simulink model "model_2_testform1"  (R2018a)
settings: Solver=VariableStepAuto  StartTime=0.0  StopTime=10.0  RelTol=1e-3
values from neighbouring files (symbols this model uses):
  Ad = [ 1   0     Tc        0 ... (first row only)    [vehicle_2DOF_model.m]    (also in vehicle_2DOF_model_2.m)
  Bd = [  0     0 ... (first row only)    [vehicle_2DOF_model.m]    (also in vehicle_2DOF_model_2.m)
  Fa = dlqr(Aa,Ba,Q,R)    [vehicle_2DOF_model.m]    (also in vehicle_2DOF_model_2.m = compute_Rstab_gain(ss(Aaug,Baug,Caug,zeros(2,2)), 2, pi/6, 5)
  Tc = 0.1    [vehicle_2DOF_model.m]    (also in vehicle_2DOF_model_2.m)
undefined symbols (not defined in the file or in its folder): DiscIntNeverNeededParam
settings Model: Creator=marwa  LastModifiedBy=marwa

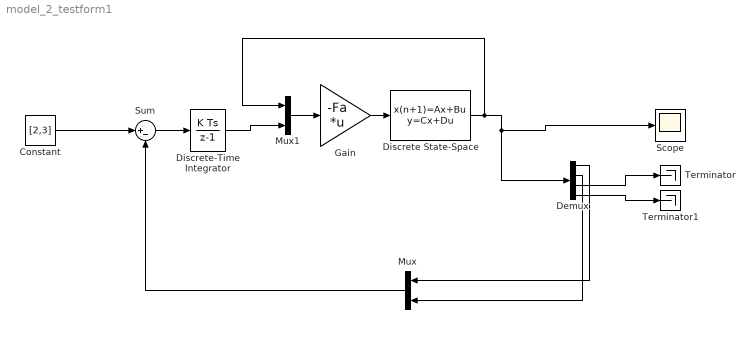
== system model_2_testform1 ==
  Constant : Constant  Value=[2,3]
  Demux : Demux
  Discrete State-Space : DiscreteStateSpace  A=Ad  B=Bd  C=eye(4)  D=zeros(4,2)  SampleTime=Tc
  Discrete-Time Integrator : DiscreteIntegrator  SampleTime=Tc  ICPrevOutput=DiscIntNeverNeededParam  ICPrevScaledInput=DiscIntNeverNeededParam
  Gain : Gain  Gain=-Fa  Multiplication=Matrix(K*u) (u vector)
  Mux : Mux  Inputs=2
  Mux1 : Mux  Inputs=2
  Scope : Scope
  Sum : Sum  Inputs=|+-
  Terminator : Terminator
  Terminator1 : Terminator
  wires:
  Constant/1 -> Sum/1
  Discrete State-Space/1 -> Mux1/1, Demux/1, Scope/1
  Sum/1 -> Discrete-Time Integrator/1
  Discrete-Time Integrator/1 -> Mux1/2
  Demux/1 -> Mux/1
  Demux/2 -> Mux/2
  Demux/3 -> Terminator/1
  Demux/4 -> Terminator1/1
  Mux/1 -> Sum/2
  Mux1/1 -> Gain/1
  Gain/1 -> Discrete State-Space/1
